simulink model "a7_real_control_pid_with_paramid"  (R2023b)
settings: Solver=FixedStepAuto  StartTime=0.0  StopTime=inf  RelTol=1e-3
undefined symbols (not defined in the file): dev, Main, pid_y_i, pwm_output0
libraries: slpidlib x12, simulink x6, px4Sensorslib x5, sharedTrackingLibrary x2, px4lib x1, px4uORBlib x1
(part 1 of 2)
settings Model: ExtModeTrigDuration=10  Creator=UAV2  LastModifiedBy=UAV2
settings SolverCC: AlgebraicLoopSolver=TrustRegion  PositivePriorityOrder=on  MaxZcPerStep=1
settings OptimizationCC: EnhancedBackFolding=on  PassReuseOutputArgsAs=Individual arguments  ZeroExternalMemoryAtStartup=off  ZeroInternalMemoryAtStartup=off  MaxStackSize=64  OptimizeBlockOrder=speed  DifferentSizesBufferReuse=on  OptimizationCustomize=off  EfficientTunableParamExpr=on
settings DebuggingCC: ParameterTunabilityLossMsg=error  UnconnectedInputMsg=warning  UnconnectedOutputMsg=warning  UnconnectedLineMsg=warning  SymbolicDimsDataTypeCodeGenerationDiagnostic=none
settings HardwareCC: ProdBitPerPointer=32  ProdBitPerSizeT=32  ProdBitPerPtrDiffT=32  ProdLargestAtomicInteger=Long  ProdLargestAtomicFloat=Double  ProdWordSize=32  ProdLongLongMode=on  ProdHWDeviceType=ARM Compatible->ARM Cortex
settings ModelReferenceCC: EnableRefExpFcnMdlSchedulingChecks=on
settings SFSimCC: SimGenImportedTypeDefs=on  MATLABDynamicMemAlloc=off  SimTargetLang=C++
settings RTWCC: Description=Embedded Coder  SystemTargetFile=ert.tlc  HardwareBoard=PX4 Pixhawk 4  TLCOptions="-aInlineSetEventsForThisBaseRateFcn=TLC_FALSE -aSuppressMultiTaskScheduler=TLC_FALSE  -aRateBasedStepFcn=0"  TemplateMakefile=ert_default_tmf  Toolchain=GNU Tools for PX4 Autopilots  IncludeHyperlinkInReport=on  TargetLang=C++  DLArmComputeVersion=19.05
settings CodeAppCC: ForceParamTrailComments=on  IgnoreCustomStorageClasses=off  OperatorAnnotations=on  SimulinkDataObjDesc=on  SFDataObjDesc=on  InsertBlockDesc=on
settings ERTTargetCC: ExtModeTransport=3  ExtModeStaticAlloc=on  ExtModeStaticAllocSize=1024  ExtModeMexFile=ext_xcp  ExtModeIntrfLevel=Level2 - Open

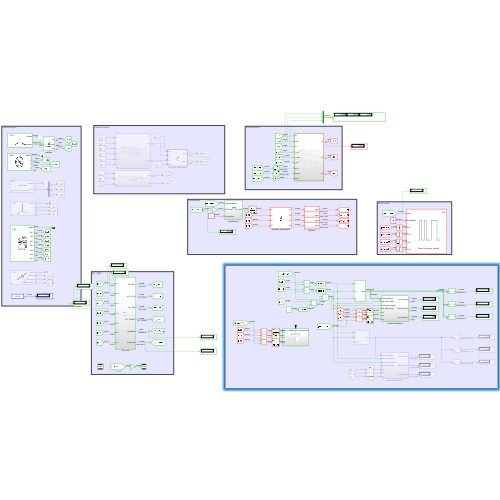
[thumbnail: Simulink's stored preview of the top-level diagram]
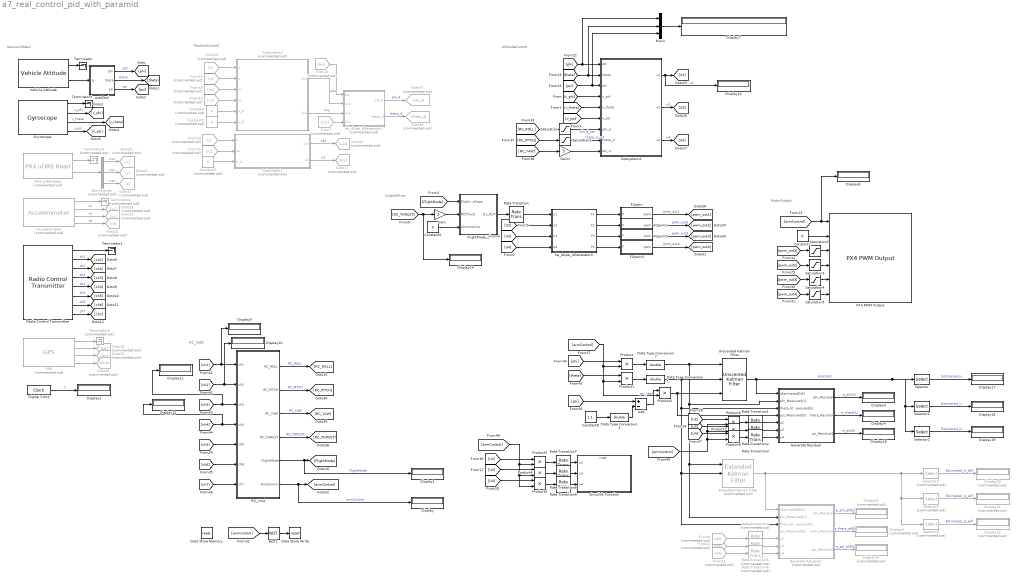
== system a7_real_control_pid_with_paramid ==
  note: RC_CMD
  note: PositionControl
  note: MotorOutput
  note: SencsorObtain
  note: AttitudeControl
  note: OutputMixer
  Accelerometer : px4Sensorslib/Accelerometer  Commented=on  uorbTimeStamp=off  BlockingMode=off  BlockTimeout=1e-3  sampleTime=1/250
  Add : Sum  Inputs=+-
  Bus Selector : BusSelector  Commented=on  OutputSignals=x,y,z
  Constant : Constant  Commented=on  Value=0
  Constant1 : Constant  Value=0  OutDataTypeStr=boolean
  Constant2 : Constant  Commented=on  Value=0
  Constant4 : Constant  Value=0  OutDataTypeStr=double
  Constant7 : Constant  Commented=on  Value=0
  Constant8 : Constant  Value=1.1  SampleTime=1/250
  Data Store Memory : DataStoreMemory  DataStoreName=reset  WriteAfterWriteMsg=warning  ShowAdditionalParam=off  OutDataTypeStr=boolean
  Data Store Write : DataStoreWrite  DataStoreName=reset  IndexOptions=Index vector (dialog)  Indices=1  OutputSizes=1
  Data Type Conversion1 : DataTypeConversion  OutDataTypeStr=double  SaturateOnIntegerOverflow=off  RndMeth=Floor
  Data Type Conversion3 : DataTypeConversion  OutDataTypeStr=double  SaturateOnIntegerOverflow=off  RndMeth=Floor
  Data Type Conversion7 : DataTypeConversion  OutDataTypeStr=double  SaturateOnIntegerOverflow=off  RndMeth=Floor
  Digital Clock : DigitalClock
  Display{,1..4,7..14,16..19} (17 alike) : Display
  Display{5..6,15,20..22} (6 alike) : Display  Commented=on
  Extended Kalman Filter : sharedTrackingLibrary/Extended Kalman Filter  Commented=on  StateTransitionFcn=uavStateFcnSimulink  HasStateTransitionJacobianFcn=off  HasAdditiveProcessNoise=Additive  ProcessNoise=0.00001  HasTimeVaryingProcessNoise=off  HasStateTransitionFcnExtraArgument=0  InitialState=[0;0;0;0;0;0;0;0;0;0.003;0.003;0.003]  InitialStateCovariance=0.00001  MeasurementFcn1=uavMeasurementFcn1  HasMeasurementJacobianFcn1=off  HasMeasurementEnablePort1=off  HasAdditiveMeasurementNoise1=Additive  MeasurementNoise1=0.00001  HasTimeVaryingMeasurementNoise1=off  HasMeasurementFcnExtraArgument1=0  HasMeasurementWrapping1=off  MeasurementFcn2=uavMeasurementFcn2  HasMeasurementJacobianFcn2=off  HasMeasurementEnablePort2=off  HasAdditiveMeasurementNoise2=Additive  MeasurementNoise2=0.00001  HasTimeVaryingMeasurementNoise2=off  HasMeasurementFcnExtraArgument2=0  HasMeasurementWrapping2=off  MeasurementFcn3=uavMeasurementFcn3  HasMeasurementJacobianFcn3=off  HasMeasurementEnablePort3=off  HasAdditiveMeasurementNoise3=Additive  MeasurementNoise3=0.00001  HasTimeVaryingMeasurementNoise3=off  HasMeasurementFcnExtraArgument3=0  HasMeasurementWrapping3=off  MeasurementFcn4=myMeasurementFcn  HasMeasurementJacobianFcn4=off  HasMeasurementEnablePort4=off  HasAdditiveMeasurementNoise4=Additive  MeasurementNoise4=1  HasTimeVaryingMeasurementNoise4=off  HasMeasurementFcnExtraArgument4=0  HasMeasurementWrapping4=off  MeasurementFcn5=myMeasurementFcn  HasMeasurementJacobianFcn5=off  HasMeasurementEnablePort5=off  HasAdditiveMeasurementNoise5=Additive  MeasurementNoise5=1  HasTimeVaryingMeasurementNoise5=off  HasMeasurementFcnExtraArgument5=0  HasMeasurementWrapping5=off  EnableMultirate=off  StateTransitionFcnSampleTime=1  MeasurementFcn1SampleTime=1  MeasurementFcn2SampleTime=1  MeasurementFcn3SampleTime=1  MeasurementFcn4SampleTime=1  MeasurementFcn5SampleTime=1  UseCurrentEstimator=on  OutputStateCovariance=off  DataType=double  SampleTime=1/250  NumberOfMeasurements=3
  F2pwm : Subsystem
  F2pwm1 : Subsystem
  F2pwm2 : Subsystem
  F2pwm3 : Subsystem
  FlightMode_z : Subsystem
  From10 : From  Commented=on  GotoTag=z
  From11 : From  Commented=on  GotoTag=U3
  From12 : From  Commented=on  GotoTag=U4
  From15 : From  Commented=on  GotoTag=x
  From16 : From  Commented=on  GotoTag=y
  From18 : From  Commented=on  GotoTag=vx
  From19 : From  Commented=on  GotoTag=vy
  From21 : From  Commented=on  GotoTag=psi
  From25 : From  Commented=on  GotoTag=vz
  From7 : From  Commented=on  GotoTag=u1z
  From8 : From  Commented=on  GotoTag=U2
  GPS : px4Sensorslib/GPS  Commented=on  lat=on  lon=on  alt=on  velocity=off  course=off  gpsfix=off  numsat=off  timestamp_utc=off  BlockingMode=off  BlockTimeout=1e-3  dop=off  vel_ned=off  alt_ellipsoid=off  jamm_ind=off  timestamp=off  sampleTime=1/250
  Gain : Gain  Gain=2
  Gain1 : Gain  Gain=3
  Generate Residual : Subsystem
  Generate Residual1 : Subsystem  Commented=on
  Goto13 : Goto  Commented=on  GotoTag=vx
  Goto14 : Goto  Commented=on  GotoTag=vy
  Goto15 : Goto  Commented=on  GotoTag=vz
  Goto17 : Goto  Commented=on  GotoTag=U1
  Goto18 : Goto  Commented=on  GotoTag=lat
  Goto19 : Goto  Commented=on  GotoTag=lon
  Goto20 : Goto  Commented=on  GotoTag=altitude
  Goto21 : Goto  Commented=on  GotoTag=x
  Goto22 : Goto  Commented=on  GotoTag=y
  Goto23 : Goto  Commented=on  GotoTag=z
  Goto24 : Goto  Commented=on  GotoTag=u1z
  Goto37 : Goto  Commented=on  GotoTag=phi_d
  Goto38 : Goto  Commented=on  GotoTag=theta_d
  Gyroscope : px4Sensorslib/Gyroscope  uorbTimeStamp=off  BlockingMode=off  BlockTimeout=1e-3  sampleTime=1/250
  Mux4 : Mux  Inputs=3
  NOT1 : Logic  Operator=NOT  IconShape=distinctive  AllPortsSameDT=off  OutDataTypeStr=boolean
  PX4 PWM Output : px4lib/PX4 PWM Output  pwmDevice=Main (/dev/pwm_output0)  pwmChannel1_=on  pwmChannel2_=on  pwmChannel3_=on  pwmChannel4_=on  pwmChannel5_=off  pwmChannel6_=off  pwmChannel7_=off  pwmChannel8_=off  forceTerminateFailsafe=off  outputErrorStatus=off
  PX4 uORB Read : px4uORBlib/PX4 uORB Read  Commented=on  uORBTopic=vehicle_local_position  selectInstance=actuator_armed  SampleTime=1/250  BlockingMode=off  BlockTimeout=1e-3
  Product{,1..8} (9 alike) : Product
  RC_cmd : Subsystem  Tag=attitudeControl
  Radio Control Transmitter : px4Sensorslib/Radio Control Transmitter  channel1=on  channel2=on  channel3=on  channel4=on  channel5=on  channel6=on  channel7=on  channel8=off  channel_count=off  rssi=off  rc_input_source=off  timestamp_last_signal=off  time_stamp=off  sampleTime=1/250  BlockingMode=off  BlockTimeout=5
  Rate Transition{,1..3,7..9} (7 alike) : RateTransition
  Rate Transition4 : RateTransition  Commented=on
  Rate Transition5 : RateTransition  Commented=on
  Rate Transition6 : RateTransition  Commented=on
  Saturation : Saturate
  Saturation1 : Saturate
  Saturation{2..5} (4 alike) : Saturate  UpperLimit=2000  LowerLimit=1050
  Selector : Selector  InputPortWidth=12  IndexOptions=Index vector (dialog)  Indices=10  OutputSizes=1
  Selector1 : Selector  InputPortWidth=12  IndexOptions=Index vector (dialog)  Indices=11  OutputSizes=1
  Selector2 : Selector  InputPortWidth=12  IndexOptions=Index vector (dialog)  Indices=12  OutputSizes=1
  Selector3 : Selector  Commented=on  InputPortWidth=12  IndexOptions=Index vector (dialog)  Indices=10  OutputSizes=1
  Selector4 : Selector  Commented=on  InputPortWidth=12  IndexOptions=Index vector (dialog)  Indices=11  OutputSizes=1
  Selector5 : Selector  Commented=on  InputPortWidth=12  IndexOptions=Index vector (dialog)  Indices=12  OutputSizes=1
  Simulink Function : Subsystem  TreatAsAtomicUnit=on
  Subsystem1 : Subsystem  Commented=on
  Subsystem3 : Subsystem  Commented=on
  Subsystem4 : Subsystem
  Terminator : Terminator
  Terminator1 : Terminator
  Terminator2 : Terminator  Commented=on
  Terminator3 : Terminator
  Terminator4 : Terminator  Commented=on
  Terminator5 : Terminator  Commented=on
  Unscented Kalman Filter : sharedTrackingLibrary/Unscented Kalman Filter  StateTransitionFcn=uavStateFcnSimulink  HasAdditiveProcessNoise=Additive  ProcessNoise=0.000000000000000000000001  HasTimeVaryingProcessNoise=off  HasStateTransitionFcnExtraArgument=0  InitialState=[0;0;0;0;0;0;0;0;0;0.003;0.003;0.003]  InitialStateCovariance=0.00001  Alpha=1e-3  Beta=2  Kappa=0  MeasurementFcn1=uavMeasurementFcn1  HasMeasurementEnablePort1=off  HasAdditiveMeasurementNoise1=Additive  MeasurementNoise1=0.000000000000000000000001  HasTimeVaryingMeasurementNoise1=off  HasMeasurementFcnExtraArgument1=0  HasMeasurementWrapping1=off  MeasurementFcn2=uavMeasurementFcn2  HasMeasurementEnablePort2=off  HasAdditiveMeasurementNoise2=Additive  MeasurementNoise2=0.000000000000000000000001  HasTimeVaryingMeasurementNoise2=off  HasMeasurementFcnExtraArgument2=0  HasMeasurementWrapping2=off  MeasurementFcn3=uavMeasurementFcn3  HasMeasurementEnablePort3=off  HasAdditiveMeasurementNoise3=Additive  MeasurementNoise3=0.000000000000000000000001  HasTimeVaryingMeasurementNoise3=off  HasMeasurementFcnExtraArgument3=0  HasMeasurementWrapping3=off  MeasurementFcn4=uavMeasurementFcn4  HasMeasurementEnablePort4=off  HasAdditiveMeasurementNoise4=Nonadditive  MeasurementNoise4=1  HasTimeVaryingMeasurementNoise4=off  HasMeasurementFcnExtraArgument4=0  HasMeasurementWrapping4=off  MeasurementFcn5=uavMeasurementFcn5  HasMeasurementEnablePort5=off  HasAdditiveMeasurementNoise5=Nonadditive  MeasurementNoise5=1  HasTimeVaryingMeasurementNoise5=off  HasMeasurementFcnExtraArgument5=0  HasMeasurementWrapping5=off  EnableMultirate=off  StateTransitionFcnSampleTime=1  MeasurementFcn1SampleTime=1  MeasurementFcn2SampleTime=1  MeasurementFcn3SampleTime=1  MeasurementFcn4SampleTime=1  MeasurementFcn5SampleTime=1  UseCurrentEstimator=on  OutputStateCovariance=off  DataType=double  SampleTime=1/250  NumberOfMeasurements=3
  Vehicle Attitude : px4Sensorslib/Vehicle Attitude  rollRate=off  pitchRate=off  yawRate=off  quaternion=on  uorbTimeStamp=off  BlockingMode=off  BlockTimeout=0.001  sampleTime=1/250
  fai_d&psi_dGenerator2 : MATLAB Function  Commented=on  TreatAsAtomicUnit=on
  fai_d&psi_dGenerator3 : MATLAB Function  TreatAsAtomicUnit=on
  quat2eul : MATLAB Function  TreatAsAtomicUnit=on
  wires:
  Mux4/1 -> Display7/1
  Accelerometer/3 -> Goto14/1  "vy"
  [v_phi] -> Subsystem4/4(v_phi)
  [armControl] -> NOT1/1
  From19/1 -> Subsystem3/4(vy)
  Constant1/1 -> PX4 PWM Output/2
  [ch3] -> Display11/1, RC_cmd/3(ch3)
  Gyroscope/3 -> [v_theta]  "v_theta"
  [ch2] -> RC_cmd/2(ch2), Display10/1
  quat2eul/2(theta) -> [theta]  "theta"
  [pwm_out3] -> Saturation4/1
  [U4] -> fai_d&psi_dGenerator3/4(u4)
  Constant2/1 -> Subsystem3/6(y_d)
  Gain/1 -> FlightMode_z/2(RCThrust)
  Constant/1 -> Subsystem3/5(x_d)
  fai_d&psi_dGenerator3/3(F3) -> F2pwm2/1(F)
  [ch6] -> RC_cmd/6(ch6)
  Bus Selector/3 -> Goto23/1  "<z>"
  [ch4] -> Display12/1, RC_cmd/4(ch4)
  FlightMode_z/1(U1_OUT) -> Rate Transition/1
  RC_cmd/5(FlightMode) -> Display1/1, [FlightMode]  "FlightMode"
  fai_d&psi_dGenerator2/2(theta_d) -> Goto38/1  "theta_d"
  Accelerometer/1 -> Terminator2/1
  Constant4/1 -> FlightMode_z/3(zControlOut)
  [v_psi] -> Subsystem4/6(v_psi)
  RC_cmd/6(ArmControl) -> Display/1, [armControl]  "armControl"
  Subsystem4/2(u3) -> [U3]  "u3"
  From16/1 -> Subsystem3/2(y)
  RC_cmd/1(RC_ROLL) -> [RC_ROLL]  "RC_ROLL"
  [RC_THRUST] -> Display14/1, Gain/1
  quat2eul/1(phi) -> [phi]  "phi"
  NOT1/1 -> Data Store Write/1
  RC_cmd/4(RC_THRUST) -> [RC_THRUST]  "RC_THRUST"
  [RC_YAW] -> Gain1/1
  [RC_ROLL] -> Saturation/1
  Vehicle Attitude/2 -> quat2eul/1(q)
  RC_cmd/2(RC_PITCH) -> [RC_PITCH]  "RC_PITCH"
  RC_cmd/3(RC_YAW) -> [RC_YAW]  "RC_YAW"
  [v_theta] -> Subsystem4/5(v_theta)
  [ch5] -> RC_cmd/5(ch5)
  F2pwm/1(pwm) -> [pwm_out1]  "pwm_out1"
  [ch7] -> RC_cmd/7(ch7)
  [pwm_out1] -> Saturation2/1
  fai_d&psi_dGenerator3/2(F2) -> F2pwm1/1(F)
  [theta] -> Mux4/2, Subsystem4/2(theta)
  [ch1] -> RC_cmd/1(ch1), Display9/1
  F2pwm1/1(pwm) -> [pwm_out2]  "pwm_out2"
  [pwm_out2] -> Saturation3/1
  Radio Control Transmitter/2 -> [ch1]  "ch1"
  fai_d&psi_dGenerator3/4(F4) -> F2pwm3/1(F)
  Accelerometer/2 -> Goto13/1  "vx"
  fai_d&psi_dGenerator3/1(F1) -> F2pwm/1(F)
  [pwm_out4] -> Saturation5/1
  Subsystem4/3(u4) -> [U4]  "u4"
  [phi] -> Mux4/1, Subsystem4/1(phi)
  Accelerometer/4 -> Goto15/1  "vz"
  Subsystem3/1(u1x) -> fai_d&psi_dGenerator2/2(u1x)  "u1x"
  Saturation1/1 -> Subsystem4/8(theta_d)  "theta_d_sat"
  Subsystem3/2(u1y) -> fai_d&psi_dGenerator2/3(u1y)  "u1y"
  From18/1 -> Subsystem3/3(vx)
  From21/1 -> fai_d&psi_dGenerator2/1(psi)
  Bus Selector/2 -> Goto22/1  "<y>"
  [psi] -> Mux4/3, Subsystem4/3(psi)
  Radio Control Transmitter/5 -> [ch4]  "ch4"
  Radio Control Transmitter/6 -> [ch5]  "ch5"
  Radio Control Transmitter/8 -> [ch7]  "ch7"
  Gyroscope/1 -> Terminator3/1
  Radio Control Transmitter/3 -> [ch2]  "ch2"
  PX4 uORB Read/2 -> Bus Selector/1
  Radio Control Transmitter/7 -> [ch6]  "ch6"
  GPS/4 -> Goto20/1
  [RC_PITCH] -> Saturation1/1
  Bus Selector/1 -> Goto21/1  "<x>"
  GPS/1 -> Terminator4/1
  From15/1 -> Subsystem3/1(x)
  quat2eul/3(psi) -> [psi]  "psi"
  Vehicle Attitude/1 -> Terminator/1
  Gyroscope/4 -> [v_psi]  "v_psi"
  F2pwm3/1(pwm) -> [pwm_out4]  "pwm_out4"
  [armControl] -> Display8/1, PX4 PWM Output/1
  Radio Control Transmitter/4 -> [ch3]  "ch3"
  Subsystem4/1(u2) -> Display13/1, [U2]  "u2"
  fai_d&psi_dGenerator2/1(phi_d) -> Goto37/1  "phi_d"
  Digital Clock/1 -> Display2/1  "t"
  GPS/2 -> Goto18/1
  Radio Control Transmitter/1 -> Terminator1/1
  PX4 uORB Read/1 -> Terminator5/1
  Saturation/1 -> Subsystem4/7(phi_d)  "phi_d_sat"
  Gyroscope/2 -> [v_phi]  "v_phi"
  GPS/3 -> Goto19/1
  F2pwm2/1(pwm) -> [pwm_out3]  "pwm_out3"
  [FlightMode] -> FlightMode_z/1(FlightModeCase)
  Saturation2/1 -> PX4 PWM Output/3
  Saturation3/1 -> PX4 PWM Output/4
  Saturation4/1 -> PX4 PWM Output/5
  Saturation5/1 -> PX4 PWM Output/6
  Rate Transition/1 -> fai_d&psi_dGenerator3/1(u1)
  [U2] -> fai_d&psi_dGenerator3/2(u2)
  [U3] -> fai_d&psi_dGenerator3/3(u3)
  Subsystem1/2(u1) -> Goto17/1  "u1"
  From10/1 -> Subsystem1/1(z)
  From25/1 -> Subsystem1/2(vz)
  Constant7/1 -> Subsystem1/3(z_d)
  Subsystem1/1(u1z) -> Goto24/1  "u1z"
  From7/1 -> fai_d&psi_dGenerator2/4(u1z)
  Gain1/1 -> Subsystem4/9(psi_d)
  Generate Residual/1(phi_Residual) -> Display3/1  "e_phi[k]"
  Generate Residual/3(psi_Residual2) -> Display16/1  "e_psi[k]"
  Unscented Kalman Filter/1 -> Selector2/1, Selector1/1, Selector/1, Generate Residual/1(xEstimated[k|k])  "xhat[k|k]"
  Extended Kalman Filter/1 -> Generate Residual1/1(xEstimated[k|k]), Selector5/1, Selector4/1, Selector3/1
  Generate Residual/2(theta_Residual) -> Display4/1  "e_theta[k]"
  Generate Residual1/2(theta_Residual) -> Display6/1  "e_theta_ekf[k]"
  From8/1 -> Rate Transition4/1
  Generate Residual1/3(psi_Residual2) -> Display15/1  "e_psi_ekf[k]"
  Selector5/1 -> Display22/1  "Estimated_Iz_ekf"
  Selector4/1 -> Display21/1  "Estimated_Iy_ekf"
  Selector3/1 -> Display20/1  "Estimated_Ix_ekf"
  Generate Residual1/1(phi_Residual) -> Display5/1  "e_phi_ekf[k]"
  From12/1 -> Rate Transition6/1
  Constant8/1 -> Data Type Conversion3/1
  From11/1 -> Rate Transition5/1
  Selector1/1 -> Display18/1  "Estimated_Iy"
  Selector2/1 -> Display19/1  "Estimated_Iz"
  Selector/1 -> Display17/1  "Estimated_Ix"
  Data Type Conversion7/1 -> Generate Residual1/2(phi_Measured[k]), Extended Kalman Filter/1, Generate Residual/2(phi_Measured[k]), Unscented Kalman Filter/1
  Data Type Conversion1/1 -> Unscented Kalman Filter/2, Generate Residual1/3(theta_Measured[k]), Extended Kalman Filter/2, Generate Residual/3(theta_Measured[k])
  [psi] -> Add/1
  Rate Transition1/1 -> Generate Residual/5(u2)
  Rate Transition2/1 -> Generate Residual/6(u3)
  Rate Transition3/1 -> Generate Residual/7(u4)
  Rate Transition6/1 -> Generate Residual1/7(u4)
  Rate Transition5/1 -> Generate Residual1/6(u3)
  Rate Transition4/1 -> Generate Residual1/5(u2)
  Rate Transition7/1 -> Simulink Function/1(u2)
  Rate Transition8/1 -> Simulink Function/2(u3)
  Rate Transition9/1 -> Simulink Function/3(u4)
  Data Type Conversion3/1 -> Add/2
  [phi] -> Product/1
  Product/1 -> Data Type Conversion7/1
  [armControl] -> Product/2, Product1/2, Product2/2
  [theta] -> Product1/1
  Product1/1 -> Data Type Conversion1/1
  Add/1 -> Product2/1  "psi_real"
  Product2/1 -> Generate Residual/4(psi_Measured[k]), Unscented Kalman Filter/3
  [U2] -> Product3/1
  Product3/1 -> Rate Transition7/1
  [armControl] -> Product4/2, Product5/2, Product3/2
  Product5/1 -> Rate Transition9/1
  Product4/1 -> Rate Transition8/1
  [U4] -> Product5/1
  [U3] -> Product4/1
  [U4] -> Product8/1
  [armControl] -> Product6/2, Product7/2, Product8/2
  [U2] -> Product6/1
  [U3] -> Product7/1
  Product6/1 -> Rate Transition1/1
  Product7/1 -> Rate Transition2/1
  Product8/1 -> Rate Transition3/1

== system a7_real_control_pid_with_paramid/F2pwm ==
  F : Inport
  Data Type Conversion : DataTypeConversion  OutDataTypeStr=uint16  SaturateOnIntegerOverflow=off  RndMeth=Floor
  F2pwmFcn : Subsystem
  Fcn : Fcn  Expr=u(1)*(1790-1050)+1050
  ThrustFactor : Constant  Value=0.3692
  pwm : Outport  OutDataTypeStr=uint16  VectorParamsAs1DForOutWhenUnconnected=off
  wires:
  F/1 -> F2pwmFcn/1(F)
  ThrustFactor/1 -> F2pwmFcn/2(ThrustFactor)
  F2pwmFcn/1(pwm) -> Fcn/1
  Fcn/1 -> Data Type Conversion/1
  Data Type Conversion/1 -> pwm/1

== system a7_real_control_pid_with_paramid/F2pwm1 ==
  F : Inport
  Data Type Conversion : DataTypeConversion  OutDataTypeStr=uint16  SaturateOnIntegerOverflow=off  RndMeth=Floor
  F2pwmFcn : Subsystem
  Fcn : Fcn  Expr=u(1)*(1790-1050)+1050
  ThrustFactor : Constant  Value=0.3692
  pwm : Outport  OutDataTypeStr=uint16  VectorParamsAs1DForOutWhenUnconnected=off
  wires:
  Data Type Conversion/1 -> pwm/1
  Fcn/1 -> Data Type Conversion/1
  F2pwmFcn/1(pwm) -> Fcn/1
  ThrustFactor/1 -> F2pwmFcn/2(ThrustFactor)
  F/1 -> F2pwmFcn/1(F)

== system a7_real_control_pid_with_paramid/F2pwm2 ==
  F : Inport
  Data Type Conversion : DataTypeConversion  OutDataTypeStr=uint16  SaturateOnIntegerOverflow=off  RndMeth=Floor
  F2pwmFcn : Subsystem
  Fcn : Fcn  Expr=u(1)*(1790-1050)+1050
  ThrustFactor : Constant  Value=0.3692
  pwm : Outport  OutDataTypeStr=uint16  VectorParamsAs1DForOutWhenUnconnected=off
  wires:
  F/1 -> F2pwmFcn/1(F)
  ThrustFactor/1 -> F2pwmFcn/2(ThrustFactor)
  F2pwmFcn/1(pwm) -> Fcn/1
  Fcn/1 -> Data Type Conversion/1
  Data Type Conversion/1 -> pwm/1

== system a7_real_control_pid_with_paramid/F2pwm3 ==
  F : Inport
  Data Type Conversion : DataTypeConversion  OutDataTypeStr=uint16  SaturateOnIntegerOverflow=off  RndMeth=Floor
  F2pwmFcn : Subsystem
  Fcn : Fcn  Expr=u(1)*(1790-1050)+1050
  ThrustFactor : Constant  Value=0.3692
  pwm : Outport  OutDataTypeStr=uint16  VectorParamsAs1DForOutWhenUnconnected=off
  wires:
  Data Type Conversion/1 -> pwm/1
  Fcn/1 -> Data Type Conversion/1
  F2pwmFcn/1(pwm) -> Fcn/1
  ThrustFactor/1 -> F2pwmFcn/2(ThrustFactor)
  F/1 -> F2pwmFcn/1(F)

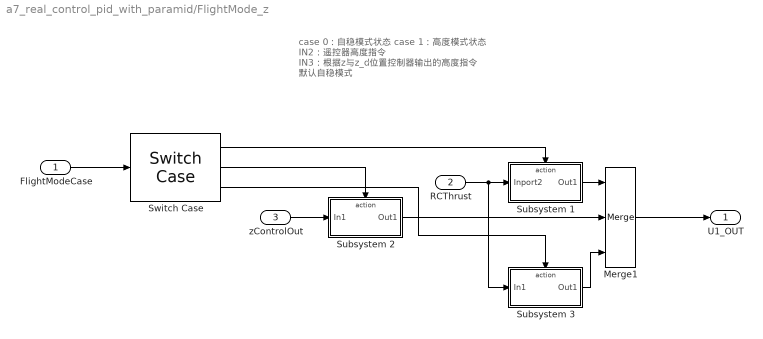
== system a7_real_control_pid_with_paramid/FlightMode_z ==
  note: case 0：自稳模式状态
      | case 1：高度模式状态
      | IN2：遥控器高度指令
      | IN3：根据z与z_d位置控制器输出的高度指令
      | 默认自稳模式
  FlightModeCase : Inport
  RCThrust : Inport  Port=2
  zControlOut : Inport  Port=3
  Merge1 : Merge  Inputs=3
  Subsystem 1 : Subsystem  TreatAsAtomicUnit=on
  Subsystem 2 : Subsystem  TreatAsAtomicUnit=on
  Subsystem 3 : Subsystem  TreatAsAtomicUnit=on
  Switch Case : SwitchCase  CaseConditions={0,1}
  U1_OUT : Outport  VectorParamsAs1DForOutWhenUnconnected=off
  wires:
  Switch Case/2 -> Subsystem 2/Action
  Subsystem 2/1(Out1) -> Merge1/2
  RCThrust/1 -> Subsystem 1/1(Inport2), Subsystem 3/1(In1)
  Switch Case/3 -> Subsystem 3/Action
  Subsystem 1/1(Out1) -> Merge1/1
  Switch Case/1 -> Subsystem 1/Action
  Subsystem 3/1(Out1) -> Merge1/3
  zControlOut/1 -> Subsystem 2/1(In1)
  FlightModeCase/1 -> Switch Case/1
  Merge1/1 -> U1_OUT/1

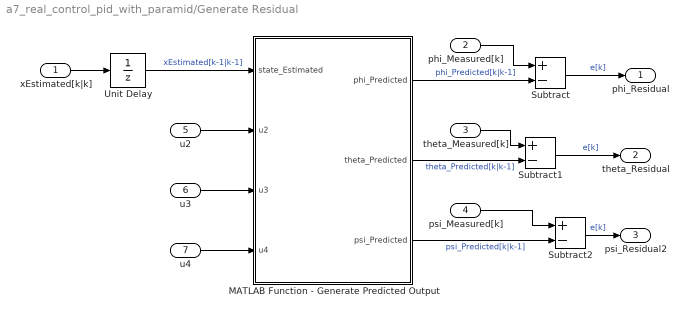
== system a7_real_control_pid_with_paramid/Generate Residual ==
  xEstimated[k|k] : Inport
  phi_Measured[k] : Inport  Port=2
  theta_Measured[k] : Inport  Port=3
  psi_Measured[k] : Inport  Port=4
  u2 : Inport  Port=5
  u3 : Inport  Port=6
  u4 : Inport  Port=7
  MATLAB Function - Generate Predicted Output : MATLAB Function  TreatAsAtomicUnit=on
  Subtract : Sum  Inputs=+-
  Subtract1 : Sum  Inputs=+-
  Subtract2 : Sum  Inputs=+-
  Unit Delay : UnitDelay  InitialCondition=[0;0;0;0;0;0;0;0;0;0.003;0.003;0.003]  SampleTime=-1  HasFrameUpgradeWarning=on
  phi_Residual : Outport  VectorParamsAs1DForOutWhenUnconnected=off
  theta_Residual : Outport  Port=2  VectorParamsAs1DForOutWhenUnconnected=off
  psi_Residual2 : Outport  Port=3  VectorParamsAs1DForOutWhenUnconnected=off
  wires:
  xEstimated[k|k]/1 -> Unit Delay/1
  Unit Delay/1 -> MATLAB Function - Generate Predicted Output/1(state_Estimated)  "xEstimated[k-1|k-1]"
  MATLAB Function - Generate Predicted Output/1(phi_Predicted) -> Subtract/2  "phi_Predicted[k|k-1]"
  Subtract/1 -> phi_Residual/1  "e[k]"
  phi_Measured[k]/1 -> Subtract/1
  MATLAB Function - Generate Predicted Output/2(theta_Predicted) -> Subtract1/2  "theta_Predicted[k|k-1]"
  Subtract1/1 -> theta_Residual/1  "e[k]"
  MATLAB Function - Generate Predicted Output/3(psi_Predicted) -> Subtract2/2  "psi_Predicted[k|k-1]"
  Subtract2/1 -> psi_Residual2/1  "e[k]"
  theta_Measured[k]/1 -> Subtract1/1
  psi_Measured[k]/1 -> Subtract2/1
  u2/1 -> MATLAB Function - Generate Predicted Output/2(u2)
  u4/1 -> MATLAB Function - Generate Predicted Output/4(u4)
  u3/1 -> MATLAB Function - Generate Predicted Output/3(u3)

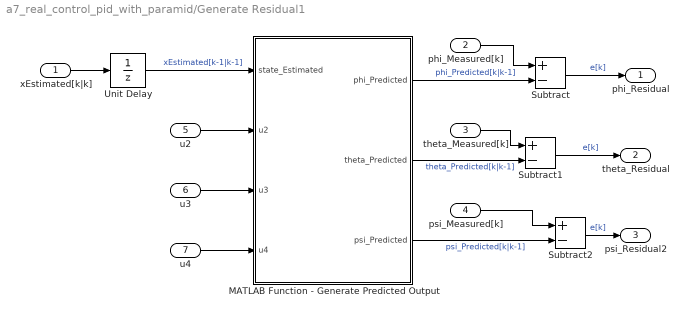
== system a7_real_control_pid_with_paramid/Generate Residual1 ==
  xEstimated[k|k] : Inport
  phi_Measured[k] : Inport  Port=2
  theta_Measured[k] : Inport  Port=3
  psi_Measured[k] : Inport  Port=4
  u2 : Inport  Port=5
  u3 : Inport  Port=6
  u4 : Inport  Port=7
  MATLAB Function - Generate Predicted Output : MATLAB Function  TreatAsAtomicUnit=on
  Subtract : Sum  Inputs=+-
  Subtract1 : Sum  Inputs=+-
  Subtract2 : Sum  Inputs=+-
  Unit Delay : UnitDelay  InitialCondition=[0;0;0;0;0;0;0;0;0;0.003;0.003;0.003]  SampleTime=-1  HasFrameUpgradeWarning=on
  phi_Residual : Outport  VectorParamsAs1DForOutWhenUnconnected=off
  theta_Residual : Outport  Port=2  VectorParamsAs1DForOutWhenUnconnected=off
  psi_Residual2 : Outport  Port=3  VectorParamsAs1DForOutWhenUnconnected=off
  wires:
  u3/1 -> MATLAB Function - Generate Predicted Output/3(u3)
  u4/1 -> MATLAB Function - Generate Predicted Output/4(u4)
  u2/1 -> MATLAB Function - Generate Predicted Output/2(u2)
  psi_Measured[k]/1 -> Subtract2/1
  theta_Measured[k]/1 -> Subtract1/1
  Subtract2/1 -> psi_Residual2/1  "e[k]"
  MATLAB Function - Generate Predicted Output/3(psi_Predicted) -> Subtract2/2  "psi_Predicted[k|k-1]"
  Subtract1/1 -> theta_Residual/1  "e[k]"
  MATLAB Function - Generate Predicted Output/2(theta_Predicted) -> Subtract1/2  "theta_Predicted[k|k-1]"
  phi_Measured[k]/1 -> Subtract/1
  Subtract/1 -> phi_Residual/1  "e[k]"
  MATLAB Function - Generate Predicted Output/1(phi_Predicted) -> Subtract/2  "phi_Predicted[k|k-1]"
  Unit Delay/1 -> MATLAB Function - Generate Predicted Output/1(state_Estimated)  "xEstimated[k-1|k-1]"
  xEstimated[k|k]/1 -> Unit Delay/1

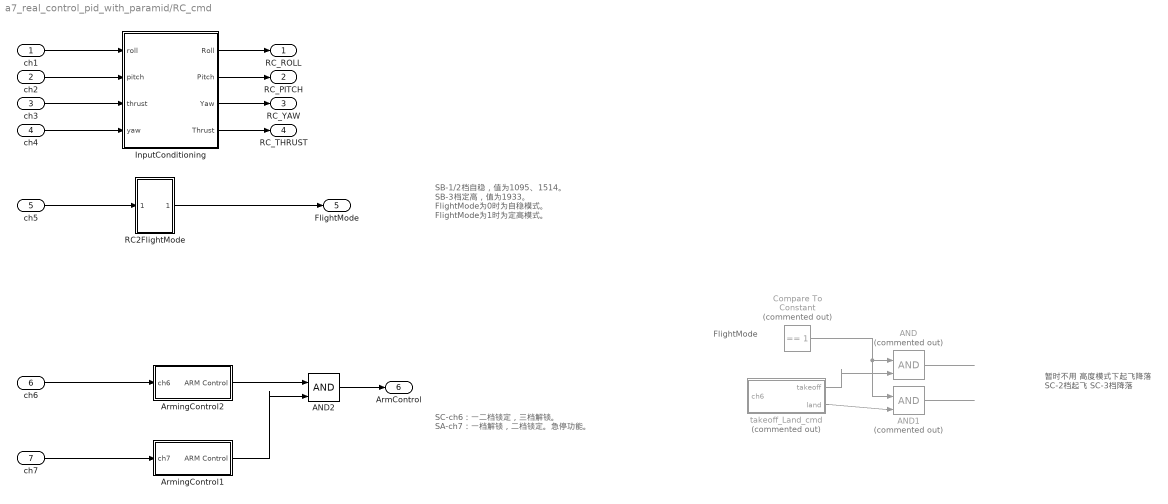
== system a7_real_control_pid_with_paramid/RC_cmd ==
  note: 暂时不用
      | 高度模式下起飞降落
      | SC-2档起飞
      | SC-3档降落
  note: SB-1/2档自稳，值为1095、1514。
      | SB-3档定高，值为1933。
      | FlightMode为0时为自稳模式。
      | FlightMode为1时为定高模式。
  note: FlightMode
  note: SC-ch6：一二档锁定，三档解锁。
      | SA-ch7：一档解锁，二档锁定。急停功能。
  ch1 : Inport  OutDataTypeStr=uint16
  ch2 : Inport  Port=2  OutDataTypeStr=uint16
  ch3 : Inport  Port=3  OutDataTypeStr=uint16
  ch4 : Inport  Port=4  OutDataTypeStr=uint16
  ch5 : Inport  Port=5  OutDataTypeStr=uint16
  ch6 : Inport  Port=6  OutDataTypeStr=uint16
  ch7 : Inport  Port=7  OutDataTypeStr=uint16
  AND : Logic  Commented=on  IconShape=distinctive  AllPortsSameDT=off  OutDataTypeStr=boolean
  AND1 : Logic  Commented=on  IconShape=distinctive  AllPortsSameDT=off  OutDataTypeStr=boolean
  AND2 : Logic  IconShape=distinctive  AllPortsSameDT=off  OutDataTypeStr=boolean
  ArmingControl1 : Subsystem
  ArmingControl2 : Subsystem
  Compare To Constant : simulink/Logic and Bit Operations/Compare To Constant  Commented=on  relop===  const=1  OutDataTypeStr=boolean
  InputConditioning : Subsystem
  RC2FlightMode : Subsystem
  takeoff_Land_cmd : Subsystem  Commented=on
  RC_ROLL : Outport
  RC_PITCH : Outport  Port=2
  RC_YAW : Outport  Port=3
  RC_THRUST : Outport  Port=4
  FlightMode : Outport  Port=5
  ArmControl : Outport  Port=6
  wires:
  ch7/1 -> ArmingControl1/1(ch7)
  ch4/1 -> InputConditioning/4(yaw)
  ch1/1 -> InputConditioning/1(roll)
  ch2/1 -> InputConditioning/2(pitch)
  ch3/1 -> InputConditioning/3(thrust)
  InputConditioning/1(Roll) -> RC_ROLL/1
  InputConditioning/2(Pitch) -> RC_PITCH/1
  InputConditioning/3(Yaw) -> RC_YAW/1
  InputConditioning/4(Thrust) -> RC_THRUST/1
  takeoff_Land_cmd/1(takeoff) -> AND/2
  AND/1 -> ?
  AND1/1 -> ?
  takeoff_Land_cmd/2(land) -> AND1/2
  ch5/1 -> RC2FlightMode/1(In1)
  RC2FlightMode/1(Out1) -> FlightMode/1
  Compare To Constant/1 -> AND1/1, AND/1
  ch6/1 -> ArmingControl2/1(ch6)
  ArmingControl2/1(ARM Control) -> AND2/1
  ArmingControl1/1(ARM Control) -> AND2/2
  AND2/1 -> ArmControl/1

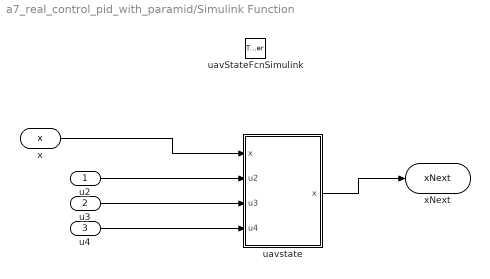
== system a7_real_control_pid_with_paramid/Simulink Function ==
  u2 : Inport
  u3 : Inport  Port=2
  u4 : Inport  Port=3
  uavStateFcnSimulink : TriggerPort  TriggerType=function-call  IsSimulinkFunction=on  FunctionName=uavStateFcnSimulink  VariantControl=Variant
  uavstate : MATLAB Function  TreatAsAtomicUnit=on
  x : ArgIn  DisableCoverage=on  PortDimensions=12  ArgumentName=x
  xNext : ArgOut  DisableCoverage=on  PortDimensions=12  ArgumentName=xNext
  wires:
  uavstate/1(x) -> xNext/1
  u2/1 -> uavstate/2(u2)
  u3/1 -> uavstate/3(u3)
  u4/1 -> uavstate/4(u4)
  x/1 -> uavstate/1("x ")

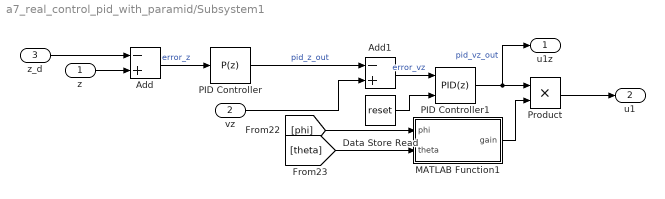
== system a7_real_control_pid_with_paramid/Subsystem1 ==
  z : Inport
  vz : Inport  Port=2
  z_d : Inport  Port=3
  Add : Sum  Inputs=-+
  Add1 : Sum  Inputs=-+
  Data Store Read : DataStoreRead  DataStoreName=reset  IndexOptions=Index vector (dialog)  Indices=1  OutputSizes=1
  MATLAB Function1 : MATLAB Function  TreatAsAtomicUnit=on
  PID Controller : slpidlib/PID Controller  Controller=P  Form=Parallel  TimeDomain=Discrete-time  UseExternalTs=off  SampleTime=-1  IntegratorMethod=Forward Euler  FilterMethod=Forward Euler  ControllerParametersSource=internal  P=1.5  I=1.33332542389365  UseKiTs=off  D=0.947452162670561  N=36.1071689779307  UseFilter=on  TunerSelectOption=Transfer Function Based (PID Tuner App)  InitialConditionSource=internal  InitialConditionForIntegrator=0  InitialConditionForFilter=0  DifferentiatorICPrevScaledInput=0  ExternalReset=none  TrackingMode=off  Kt=1  LimitOutput=on  SatLimitsSource=internal  UpperSaturationLimit=10  LowerSaturationLimit=-10  LinearizeAsGain=off  AntiWindupMode=none  Kb=1  LimitIntegrator=off  UpperIntegratorSaturationLimit=inf  LowerIntegratorSaturationLimit=-inf  POutMin=[]  POutMax=[]  IOutMin=[]  IOutMax=[]  DOutMin=[]  DOutMax=[]  NOutMin=[]  NOutMax=[]  SumOutMin=[]  SumOutMax=[]  SaturationOutMin=[]  SaturationOutMax=[]  PParamMin=[]  PParamMax=[]  IParamMin=[]  IParamMax=[]  DParamMin=[]  DParamMax=[]  NParamMin=[]  NParamMax=[]  KbParamMin=[]  KbParamMax=[]  KtParamMin=[]  KtParamMax=[]  KbOutMin=[]  KbOutMax=[]  KtOutMin=[]  KtOutMax=[]  IntegratorOutMin=[]  IntegratorOutMax=[]  FilterOutMin=[]  FilterOutMax=[]  SumI1OutMin=[]  SumI1OutMax=[]  SumI2OutMin=[]  SumI2OutMax=[]  SumI3OutMin=[]  SumI3OutMax=[]  SumI4OutMin=[]  SumI4OutMax=[]  SumDOutMin=[]  SumDOutMax=[]  DifferentiatorOutMin=[]  DifferentiatorOutMax=[]  FilterDiffOutCoefMin=[]  FilterDiffOutCoefMax=[]  ReciprocalOutMin=[]  ReciprocalOutMax=[]  SumDenOutMin=[]  SumDenOutMax=[]  SumNumOutMin=[]  SumNumOutMax=[]  DivideOutMin=[]  DivideOutMax=[]  UdiffTsProdOutMin=[]  UdiffTsProdOutMax=[]  NTsProdOutMin=[]  NTsProdOutMax=[]  UintegralTsProdOutMin=[]  UintegralTsProdOutMax=[]  UngainTsProdOutMin=[]  UngainTsProdOutMax=[]  ClampingZeroOutDataTypeStr=Inherit: Inherit via back propagation  ClampingZeroOutMin=[]  ClampingZeroOutMax=[]  FilterDenConstantOutDataTypeStr=Inherit: Inherit via back propagation  FilterDenConstantOutMin=[]  FilterDenConstantOutMax=[]  PCopyOutDataTypeStr=Inherit: Inherit via back propagation  PCopyOutMin=[]  PCopyOutMax=[]  NCopyOutDataTypeStr=Inherit: Inherit via back propagation  NCopyOutMin=[]  NCopyOutMax=[]  IntegratorContinuousStateAttributes=''  IntegratorStateMustResolveToSignalObject=off  IntegratorRTWStateStorageClass=Auto  FilterContinuousStateAttributes=''  FilterStateMustResolveToSignalObject=off  FilterRTWStateStorageClass=Auto  ParallelPVariant=InternalParameters  IdealPVariant=Disabled  IVariant=Disabled  DVariant=Disabled  IntegratorVariant=Disabled  SatVariant=Enabled  AWVariant=Disabled  PCopyVariant=Disabled  TRVariant=Disabled  FdbkBlocksVariant=Forward  IdealPFdbkVariant=Disabled  SatFdbkVariant=Disabled  DerivativeFilterVariant=Disabled  NVariant=Disabled  NCopyVariant=Disabled_SignalSpec  FilterICVariant=Disabled  IntegratorICVariant=Disabled  ExternalResetVariant=Disabled  TRSumVariant=Passthrough  SumFdbkVariant=Disabled  SumVariant=Passthrough_P  TsampFilterVariant=InternalTs  TsampNgainVariant=Passthrough  TsampIntegralVariant=Disabled_SignalSpec  ExternalSaturationOutDataTypeStr=Inherit: Same as second input
  PID Controller1 : slpidlib/PID Controller  Controller=PID  Form=Parallel  TimeDomain=Discrete-time  UseExternalTs=off  SampleTime=-1  IntegratorMethod=Forward Euler  FilterMethod=Forward Euler  ControllerParametersSource=internal  P=0.6  I=0.3  UseKiTs=off  D=0  N=10  UseFilter=on  TunerSelectOption=Transfer Function Based (PID Tuner App)  InitialConditionSource=internal  InitialConditionForIntegrator=0  InitialConditionForFilter=0  DifferentiatorICPrevScaledInput=0  ExternalReset=level  TrackingMode=off  Kt=1  LimitOutput=on  SatLimitsSource=internal  UpperSaturationLimit=1  LowerSaturationLimit=0  LinearizeAsGain=off  AntiWindupMode=none  Kb=1  LimitIntegrator=off  UpperIntegratorSaturationLimit=0.1  LowerIntegratorSaturationLimit=-0.1  POutMin=[]  POutMax=[]  IOutMin=[]  IOutMax=[]  DOutMin=[]  DOutMax=[]  NOutMin=[]  NOutMax=[]  SumOutMin=[]  SumOutMax=[]  SaturationOutMin=[]  SaturationOutMax=[]  PParamMin=[]  PParamMax=[]  IParamMin=[]  IParamMax=[]  DParamMin=[]  DParamMax=[]  NParamMin=[]  NParamMax=[]  KbParamMin=[]  KbParamMax=[]  KtParamMin=[]  KtParamMax=[]  KbOutMin=[]  KbOutMax=[]  KtOutMin=[]  KtOutMax=[]  IntegratorOutMin=[]  IntegratorOutMax=[]  FilterOutMin=[]  FilterOutMax=[]  SumI1OutMin=[]  SumI1OutMax=[]  SumI2OutMin=[]  SumI2OutMax=[]  SumI3OutMin=[]  SumI3OutMax=[]  SumI4OutMin=[]  SumI4OutMax=[]  SumDOutMin=[]  SumDOutMax=[]  DifferentiatorOutMin=[]  DifferentiatorOutMax=[]  FilterDiffOutCoefMin=[]  FilterDiffOutCoefMax=[]  ReciprocalOutMin=[]  ReciprocalOutMax=[]  SumDenOutMin=[]  SumDenOutMax=[]  SumNumOutMin=[]  SumNumOutMax=[]  DivideOutMin=[]  DivideOutMax=[]  UdiffTsProdOutMin=[]  UdiffTsProdOutMax=[]  NTsProdOutMin=[]  NTsProdOutMax=[]  UintegralTsProdOutMin=[]  UintegralTsProdOutMax=[]  UngainTsProdOutMin=[]  UngainTsProdOutMax=[]  ClampingZeroOutDataTypeStr=Inherit: Inherit via back propagation  ClampingZeroOutMin=[]  ClampingZeroOutMax=[]  FilterDenConstantOutDataTypeStr=Inherit: Inherit via back propagation  FilterDenConstantOutMin=[]  FilterDenConstantOutMax=[]  PCopyOutDataTypeStr=Inherit: Inherit via back propagation  PCopyOutMin=[]  PCopyOutMax=[]  NCopyOutDataTypeStr=Inherit: Inherit via back propagation  NCopyOutMin=[]  NCopyOutMax=[]  IntegratorContinuousStateAttributes=''  IntegratorStateMustResolveToSignalObject=off  IntegratorRTWStateStorageClass=Auto  FilterContinuousStateAttributes=''  FilterStateMustResolveToSignalObject=off  FilterRTWStateStorageClass=Auto  ParallelPVariant=InternalParameters  IdealPVariant=Disabled  IVariant=InternalParameters  DVariant=InternalParameters  IntegratorVariant=Discrete  SatVariant=Enabled  AWVariant=Passthrough  PCopyVariant=Disabled  TRVariant=Disabled  FdbkBlocksVariant=Forward  IdealPFdbkVariant=Disabled  SatFdbkVariant=Disabled  DerivativeFilterVariant=ForwardEulerFilter  NVariant=InternalParameters  NCopyVariant=Disabled  FilterICVariant=InternalICsFilter  IntegratorICVariant=InternalICs  ExternalResetVariant=ExternalReset  TRSumVariant=Passthrough  SumFdbkVariant=Disabled  SumVariant=Sum_PID  TsampFilterVariant=InternalTs  TsampNgainVariant=Passthrough  TsampIntegralVariant=Disabled_SignalSpec  ExternalSaturationOutDataTypeStr=Inherit: Same as second input
  Product : Product
  u1z : Outport
  u1 : Outport  Port=2
  wires:
  z/1 -> Add/2
  z_d/1 -> Add/1
  Data Store Read/1 -> PID Controller1/2
  Add1/1 -> PID Controller1/1  "error_vz"
  PID Controller/1 -> Add1/1  "pid_z_out"
  PID Controller1/1 -> Product/1, u1z/1  "pid_vz_out"
  vz/1 -> Add1/2
  MATLAB Function1/1(gain) -> Product/2
  [theta] -> MATLAB Function1/2(theta)
  Product/1 -> u1/1
  Add/1 -> PID Controller/1  "error_z"
  [phi] -> MATLAB Function1/1(phi)

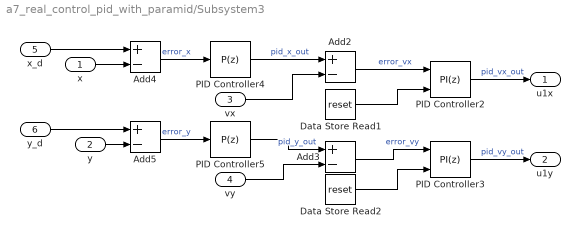
== system a7_real_control_pid_with_paramid/Subsystem3 ==
  x : Inport
  y : Inport  Port=2
  vx : Inport  Port=3
  vy : Inport  Port=4
  x_d : Inport  Port=5
  y_d : Inport  Port=6
  Add{2..5} (4 alike) : Sum  Inputs=+-
  Data Store Read1 : DataStoreRead  DataStoreName=reset  IndexOptions=Index vector (dialog)  Indices=1  OutputSizes=1
  Data Store Read2 : DataStoreRead  DataStoreName=reset  IndexOptions=Index vector (dialog)  Indices=1  OutputSizes=1
  PID Controller2 : slpidlib/PID Controller  Controller=PI  Form=Parallel  TimeDomain=Discrete-time  UseExternalTs=off  SampleTime=-1  IntegratorMethod=Forward Euler  FilterMethod=Forward Euler  ControllerParametersSource=internal  P=0.1  I=0.01  UseKiTs=off  D=0.947452162670561  N=36.1071689779307  UseFilter=on  TunerSelectOption=Transfer Function Based (PID Tuner App)  InitialConditionSource=internal  InitialConditionForIntegrator=0  InitialConditionForFilter=0  DifferentiatorICPrevScaledInput=0  ExternalReset=level  TrackingMode=off  Kt=1  LimitOutput=on  SatLimitsSource=internal  UpperSaturationLimit=1  LowerSaturationLimit=-1  LinearizeAsGain=off  AntiWindupMode=none  Kb=1  LimitIntegrator=off  UpperIntegratorSaturationLimit=inf  LowerIntegratorSaturationLimit=-inf  POutMin=[]  POutMax=[]  IOutMin=[]  IOutMax=[]  DOutMin=[]  DOutMax=[]  NOutMin=[]  NOutMax=[]  SumOutMin=[]  SumOutMax=[]  SaturationOutMin=[]  SaturationOutMax=[]  PParamMin=[]  PParamMax=[]  IParamMin=[]  IParamMax=[]  DParamMin=[]  DParamMax=[]  NParamMin=[]  NParamMax=[]  KbParamMin=[]  KbParamMax=[]  KtParamMin=[]  KtParamMax=[]  KbOutMin=[]  KbOutMax=[]  KtOutMin=[]  KtOutMax=[]  IntegratorOutMin=[]  IntegratorOutMax=[]  FilterOutMin=[]  FilterOutMax=[]  SumI1OutMin=[]  SumI1OutMax=[]  SumI2OutMin=[]  SumI2OutMax=[]  SumI3OutMin=[]  SumI3OutMax=[]  SumI4OutMin=[]  SumI4OutMax=[]  SumDOutMin=[]  SumDOutMax=[]  DifferentiatorOutMin=[]  DifferentiatorOutMax=[]  FilterDiffOutCoefMin=[]  FilterDiffOutCoefMax=[]  ReciprocalOutMin=[]  ReciprocalOutMax=[]  SumDenOutMin=[]  SumDenOutMax=[]  SumNumOutMin=[]  SumNumOutMax=[]  DivideOutMin=[]  DivideOutMax=[]  UdiffTsProdOutMin=[]  UdiffTsProdOutMax=[]  NTsProdOutMin=[]  NTsProdOutMax=[]  UintegralTsProdOutMin=[]  UintegralTsProdOutMax=[]  UngainTsProdOutMin=[]  UngainTsProdOutMax=[]  ClampingZeroOutDataTypeStr=Inherit: Inherit via back propagation  ClampingZeroOutMin=[]  ClampingZeroOutMax=[]  FilterDenConstantOutDataTypeStr=Inherit: Inherit via back propagation  FilterDenConstantOutMin=[]  FilterDenConstantOutMax=[]  PCopyOutDataTypeStr=Inherit: Inherit via back propagation  PCopyOutMin=[]  PCopyOutMax=[]  NCopyOutDataTypeStr=Inherit: Inherit via back propagation  NCopyOutMin=[]  NCopyOutMax=[]  IntegratorContinuousStateAttributes=''  IntegratorStateMustResolveToSignalObject=off  IntegratorRTWStateStorageClass=Auto  FilterContinuousStateAttributes=''  FilterStateMustResolveToSignalObject=off  FilterRTWStateStorageClass=Auto  ParallelPVariant=InternalParameters  IdealPVariant=Disabled  IVariant=InternalParameters  DVariant=Disabled  IntegratorVariant=Discrete  SatVariant=Enabled  AWVariant=Passthrough  PCopyVariant=Disabled  TRVariant=Disabled  FdbkBlocksVariant=Forward  IdealPFdbkVariant=Disabled  SatFdbkVariant=Disabled  DerivativeFilterVariant=Disabled  NVariant=Disabled  NCopyVariant=Disabled_SignalSpec  FilterICVariant=Disabled  IntegratorICVariant=InternalICs  ExternalResetVariant=ExternalReset  TRSumVariant=Passthrough  SumFdbkVariant=Disabled  SumVariant=Sum_PI  TsampFilterVariant=InternalTs  TsampNgainVariant=Passthrough  TsampIntegralVariant=Disabled_SignalSpec  ExternalSaturationOutDataTypeStr=Inherit: Same as second input
  PID Controller3 : slpidlib/PID Controller  Controller=PI  Form=Parallel  TimeDomain=Discrete-time  UseExternalTs=off  SampleTime=-1  IntegratorMethod=Forward Euler  FilterMethod=Forward Euler  ControllerParametersSource=internal  P=0.1  I=0.01  UseKiTs=off  D=0  N=10  UseFilter=off  TunerSelectOption=Transfer Function Based (PID Tuner App)  InitialConditionSource=internal  InitialConditionForIntegrator=0  InitialConditionForFilter=0  DifferentiatorICPrevScaledInput=0  ExternalReset=level  TrackingMode=off  Kt=1  LimitOutput=on  SatLimitsSource=internal  UpperSaturationLimit=1  LowerSaturationLimit=-1  LinearizeAsGain=off  AntiWindupMode=none  Kb=1  LimitIntegrator=off  UpperIntegratorSaturationLimit=inf  LowerIntegratorSaturationLimit=-inf  POutMin=[]  POutMax=[]  IOutMin=[]  IOutMax=[]  DOutMin=[]  DOutMax=[]  NOutMin=[]  NOutMax=[]  SumOutMin=[]  SumOutMax=[]  SaturationOutMin=[]  SaturationOutMax=[]  PParamMin=[]  PParamMax=[]  IParamMin=[]  IParamMax=[]  DParamMin=[]  DParamMax=[]  NParamMin=[]  NParamMax=[]  KbParamMin=[]  KbParamMax=[]  KtParamMin=[]  KtParamMax=[]  KbOutMin=[]  KbOutMax=[]  KtOutMin=[]  KtOutMax=[]  IntegratorOutMin=[]  IntegratorOutMax=[]  FilterOutMin=[]  FilterOutMax=[]  SumI1OutMin=[]  SumI1OutMax=[]  SumI2OutMin=[]  SumI2OutMax=[]  SumI3OutMin=[]  SumI3OutMax=[]  SumI4OutMin=[]  SumI4OutMax=[]  SumDOutMin=[]  SumDOutMax=[]  DifferentiatorOutMin=[]  DifferentiatorOutMax=[]  FilterDiffOutCoefMin=[]  FilterDiffOutCoefMax=[]  ReciprocalOutMin=[]  ReciprocalOutMax=[]  SumDenOutMin=[]  SumDenOutMax=[]  SumNumOutMin=[]  SumNumOutMax=[]  DivideOutMin=[]  DivideOutMax=[]  UdiffTsProdOutMin=[]  UdiffTsProdOutMax=[]  NTsProdOutMin=[]  NTsProdOutMax=[]  UintegralTsProdOutMin=[]  UintegralTsProdOutMax=[]  UngainTsProdOutMin=[]  UngainTsProdOutMax=[]  ClampingZeroOutDataTypeStr=Inherit: Inherit via back propagation  ClampingZeroOutMin=[]  ClampingZeroOutMax=[]  FilterDenConstantOutDataTypeStr=Inherit: Inherit via back propagation  FilterDenConstantOutMin=[]  FilterDenConstantOutMax=[]  PCopyOutDataTypeStr=Inherit: Inherit via back propagation  PCopyOutMin=[]  PCopyOutMax=[]  NCopyOutDataTypeStr=Inherit: Inherit via back propagation  NCopyOutMin=[]  NCopyOutMax=[]  IntegratorContinuousStateAttributes=''  IntegratorStateMustResolveToSignalObject=off  IntegratorRTWStateStorageClass=Auto  FilterContinuousStateAttributes=''  FilterStateMustResolveToSignalObject=off  FilterRTWStateStorageClass=Auto  ParallelPVariant=InternalParameters  IdealPVariant=Disabled  IVariant=InternalParameters  DVariant=Disabled  IntegratorVariant=Discrete  SatVariant=Enabled  AWVariant=Passthrough  PCopyVariant=Disabled  TRVariant=Disabled  FdbkBlocksVariant=Forward  IdealPFdbkVariant=Disabled  SatFdbkVariant=Disabled  DerivativeFilterVariant=Disabled  NVariant=Disabled  NCopyVariant=Disabled_SignalSpec  FilterICVariant=Disabled  IntegratorICVariant=InternalICs  ExternalResetVariant=ExternalReset  TRSumVariant=Passthrough  SumFdbkVariant=Disabled  SumVariant=Sum_PI  TsampFilterVariant=InternalTs  TsampNgainVariant=Passthrough  TsampIntegralVariant=Disabled_SignalSpec  ExternalSaturationOutDataTypeStr=Inherit: Same as second input
  PID Controller4 : slpidlib/PID Controller  Controller=P  Form=Parallel  TimeDomain=Discrete-time  UseExternalTs=off  SampleTime=-1  IntegratorMethod=Forward Euler  FilterMethod=Forward Euler  ControllerParametersSource=internal  P=0.8  I=0.02  UseKiTs=off  D=0.245723815521348  N=312.971612169429  UseFilter=on  TunerSelectOption=Transfer Function Based (PID Tuner App)  InitialConditionSource=internal  InitialConditionForIntegrator=0  InitialConditionForFilter=0  DifferentiatorICPrevScaledInput=0  ExternalReset=none  TrackingMode=off  Kt=1  LimitOutput=on  SatLimitsSource=internal  UpperSaturationLimit=10  LowerSaturationLimit=-10  LinearizeAsGain=off  AntiWindupMode=none  Kb=1  LimitIntegrator=off  UpperIntegratorSaturationLimit=inf  LowerIntegratorSaturationLimit=-inf  POutMin=[]  POutMax=[]  IOutMin=[]  IOutMax=[]  DOutMin=[]  DOutMax=[]  NOutMin=[]  NOutMax=[]  SumOutMin=[]  SumOutMax=[]  SaturationOutMin=[]  SaturationOutMax=[]  PParamMin=[]  PParamMax=[]  IParamMin=[]  IParamMax=[]  DParamMin=[]  DParamMax=[]  NParamMin=[]  NParamMax=[]  KbParamMin=[]  KbParamMax=[]  KtParamMin=[]  KtParamMax=[]  KbOutMin=[]  KbOutMax=[]  KtOutMin=[]  KtOutMax=[]  IntegratorOutMin=[]  IntegratorOutMax=[]  FilterOutMin=[]  FilterOutMax=[]  SumI1OutMin=[]  SumI1OutMax=[]  SumI2OutMin=[]  SumI2OutMax=[]  SumI3OutMin=[]  SumI3OutMax=[]  SumI4OutMin=[]  SumI4OutMax=[]  SumDOutMin=[]  SumDOutMax=[]  DifferentiatorOutMin=[]  DifferentiatorOutMax=[]  FilterDiffOutCoefMin=[]  FilterDiffOutCoefMax=[]  ReciprocalOutMin=[]  ReciprocalOutMax=[]  SumDenOutMin=[]  SumDenOutMax=[]  SumNumOutMin=[]  SumNumOutMax=[]  DivideOutMin=[]  DivideOutMax=[]  UdiffTsProdOutMin=[]  UdiffTsProdOutMax=[]  NTsProdOutMin=[]  NTsProdOutMax=[]  UintegralTsProdOutMin=[]  UintegralTsProdOutMax=[]  UngainTsProdOutMin=[]  UngainTsProdOutMax=[]  ClampingZeroOutDataTypeStr=Inherit: Inherit via back propagation  ClampingZeroOutMin=[]  ClampingZeroOutMax=[]  FilterDenConstantOutDataTypeStr=Inherit: Inherit via back propagation  FilterDenConstantOutMin=[]  FilterDenConstantOutMax=[]  PCopyOutDataTypeStr=Inherit: Inherit via back propagation  PCopyOutMin=[]  PCopyOutMax=[]  NCopyOutDataTypeStr=Inherit: Inherit via back propagation  NCopyOutMin=[]  NCopyOutMax=[]  IntegratorContinuousStateAttributes=''  IntegratorStateMustResolveToSignalObject=off  IntegratorRTWStateStorageClass=Auto  FilterContinuousStateAttributes=''  FilterStateMustResolveToSignalObject=off  FilterRTWStateStorageClass=Auto  ParallelPVariant=InternalParameters  IdealPVariant=Disabled  IVariant=Disabled  DVariant=Disabled  IntegratorVariant=Disabled  SatVariant=Enabled  AWVariant=Disabled  PCopyVariant=Disabled  TRVariant=Disabled  FdbkBlocksVariant=Forward  IdealPFdbkVariant=Disabled  SatFdbkVariant=Disabled  DerivativeFilterVariant=Disabled  NVariant=Disabled  NCopyVariant=Disabled_SignalSpec  FilterICVariant=Disabled  IntegratorICVariant=Disabled  ExternalResetVariant=Disabled  TRSumVariant=Passthrough  SumFdbkVariant=Disabled  SumVariant=Passthrough_P  TsampFilterVariant=InternalTs  TsampNgainVariant=Passthrough  TsampIntegralVariant=Disabled_SignalSpec  ExternalSaturationOutDataTypeStr=Inherit: Same as second input
  PID Controller5 : slpidlib/PID Controller  Controller=P  Form=Parallel  TimeDomain=Discrete-time  UseExternalTs=off  SampleTime=-1  IntegratorMethod=Forward Euler  FilterMethod=Forward Euler  ControllerParametersSource=internal  P=0.8  I=pid_y_i  UseKiTs=off  D=0.377572647695254  N=483.906486380362  UseFilter=on  TunerSelectOption=Transfer Function Based (PID Tuner App)  InitialConditionSource=internal  InitialConditionForIntegrator=0  InitialConditionForFilter=0  DifferentiatorICPrevScaledInput=0  ExternalReset=none  TrackingMode=off  Kt=1  LimitOutput=on  SatLimitsSource=internal  UpperSaturationLimit=10  LowerSaturationLimit=-10  LinearizeAsGain=off  AntiWindupMode=none  Kb=1  LimitIntegrator=off  UpperIntegratorSaturationLimit=inf  LowerIntegratorSaturationLimit=-inf  POutMin=[]  POutMax=[]  IOutMin=[]  IOutMax=[]  DOutMin=[]  DOutMax=[]  NOutMin=[]  NOutMax=[]  SumOutMin=[]  SumOutMax=[]  SaturationOutMin=[]  SaturationOutMax=[]  PParamMin=[]  PParamMax=[]  IParamMin=[]  IParamMax=[]  DParamMin=[]  DParamMax=[]  NParamMin=[]  NParamMax=[]  KbParamMin=[]  KbParamMax=[]  KtParamMin=[]  KtParamMax=[]  KbOutMin=[]  KbOutMax=[]  KtOutMin=[]  KtOutMax=[]  IntegratorOutMin=[]  IntegratorOutMax=[]  FilterOutMin=[]  FilterOutMax=[]  SumI1OutMin=[]  SumI1OutMax=[]  SumI2OutMin=[]  SumI2OutMax=[]  SumI3OutMin=[]  SumI3OutMax=[]  SumI4OutMin=[]  SumI4OutMax=[]  SumDOutMin=[]  SumDOutMax=[]  DifferentiatorOutMin=[]  DifferentiatorOutMax=[]  FilterDiffOutCoefMin=[]  FilterDiffOutCoefMax=[]  ReciprocalOutMin=[]  ReciprocalOutMax=[]  SumDenOutMin=[]  SumDenOutMax=[]  SumNumOutMin=[]  SumNumOutMax=[]  DivideOutMin=[]  DivideOutMax=[]  UdiffTsProdOutMin=[]  UdiffTsProdOutMax=[]  NTsProdOutMin=[]  NTsProdOutMax=[]  UintegralTsProdOutMin=[]  UintegralTsProdOutMax=[]  UngainTsProdOutMin=[]  UngainTsProdOutMax=[]  ClampingZeroOutDataTypeStr=Inherit: Inherit via back propagation  ClampingZeroOutMin=[]  ClampingZeroOutMax=[]  FilterDenConstantOutDataTypeStr=Inherit: Inherit via back propagation  FilterDenConstantOutMin=[]  FilterDenConstantOutMax=[]  PCopyOutDataTypeStr=Inherit: Inherit via back propagation  PCopyOutMin=[]  PCopyOutMax=[]  NCopyOutDataTypeStr=Inherit: Inherit via back propagation  NCopyOutMin=[]  NCopyOutMax=[]  IntegratorContinuousStateAttributes=''  IntegratorStateMustResolveToSignalObject=off  IntegratorRTWStateStorageClass=Auto  FilterContinuousStateAttributes=''  FilterStateMustResolveToSignalObject=off  FilterRTWStateStorageClass=Auto  ParallelPVariant=InternalParameters  IdealPVariant=Disabled  IVariant=Disabled  DVariant=Disabled  IntegratorVariant=Disabled  SatVariant=Enabled  AWVariant=Disabled  PCopyVariant=Disabled  TRVariant=Disabled  FdbkBlocksVariant=Forward  IdealPFdbkVariant=Disabled  SatFdbkVariant=Disabled  DerivativeFilterVariant=Disabled  NVariant=Disabled  NCopyVariant=Disabled_SignalSpec  FilterICVariant=Disabled  IntegratorICVariant=Disabled  ExternalResetVariant=Disabled  TRSumVariant=Passthrough  SumFdbkVariant=Disabled  SumVariant=Passthrough_P  TsampFilterVariant=InternalTs  TsampNgainVariant=Passthrough  TsampIntegralVariant=Disabled_SignalSpec  ExternalSaturationOutDataTypeStr=Inherit: Same as second input
  u1x : Outport
  u1y : Outport  Port=2
  wires:
  PID Controller5/1 -> Add3/1  "pid_y_out"
  Data Store Read2/1 -> PID Controller3/2
  x_d/1 -> Add4/1
  PID Controller3/1 -> u1y/1  "pid_vy_out"
  Add4/1 -> PID Controller4/1  "error_x"
  vy/1 -> Add3/2
  vx/1 -> Add2/2
  PID Controller4/1 -> Add2/1  "pid_x_out"
  Add3/1 -> PID Controller3/1  "error_vy"
  PID Controller2/1 -> u1x/1  "pid_vx_out"
  Add2/1 -> PID Controller2/1  "error_vx"
  Add5/1 -> PID Controller5/1  "error_y"
  y_d/1 -> Add5/1
  Data Store Read1/1 -> PID Controller2/2
  x/1 -> Add4/2
  y/1 -> Add5/2
